simulink model "Q2_B"  (R2021a)
settings: Solver=VariableStepAuto  StartTime=0.0  StopTime=10.0  RelTol=1e-3
undefined symbols (not defined in the file or in its folder): B
settings Model: Creator=Mohammad  LastModifiedBy=Mohammad

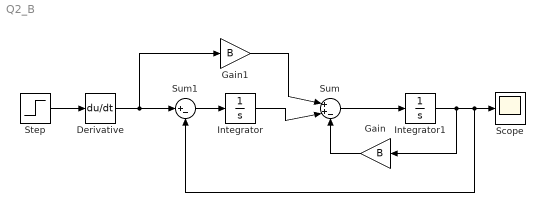
== system Q2_B ==
  Derivative : Derivative
  Gain : Gain  Gain=B
  Gain1 : Gain  Gain=B
  Integrator : Integrator
  Integrator1 : Integrator
  Scope : Scope
  Step : Step  Time=0.001  SampleTime=0
  Sum : Sum  Inputs=|++-
  Sum1 : Sum  Inputs=|+-
  wires:
  Gain/1 -> Sum/3
  Integrator1/1 -> Sum1/2, Scope/1, Gain/1
  Gain1/1 -> Sum/1
  Integrator/1 -> Sum/2
  Sum1/1 -> Integrator/1
  Step/1 -> Derivative/1
  Derivative/1 -> Gain1/1, Sum1/1
  Sum/1 -> Integrator1/1
